simulink model "adc_sample"  (Simulink 8.3)
settings: Solver=ode5  StartTime=0.0  StopTime=3  FixedStep=1/20000  RelTol=1e-3
libraries: dsparch4 x2
settings Model: Creator=hlzhang  LastModifiedBy=hlzhang
settings DataIOCC: SignalLoggingName=sigsOut
settings DebuggingCC: SaveWithParameterizedLinksMsg=none  SignalResolutionControl=TryResolveAllWithWarning  SolverPrmCheckMsg=none  MultiTaskDSMMsg=warning  MultiTaskCondExecSysMsg=none  StateNameClashWarn=none
settings HardwareCC: TargetUnknown=on
settings RTWCC: IncludeERTFirstTime=on

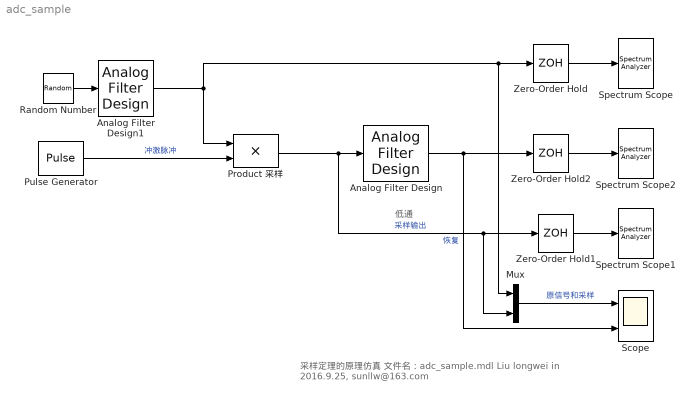
== system adc_sample ==
  note: 低通
  note: 采样定理的原理仿真
      | 文件名：adc_sample.mdl
      | Liu longwei in 2016.9.25, sunllw@163.com
  Analog Filter Design : dsparch4/Analog Filter Design  method=Butterworth  filttype=Lowpass  N=8  Wlo=2*pi*200  Whi=80  Rp=2  Rs=40
  Analog Filter Design1 : dsparch4/Analog Filter Design  method=Butterworth  filttype=Lowpass  N=50  Wlo=2*pi*250  Whi=80  Rp=2  Rs=40
  Mux : Mux  Inputs=2
  Product 采样 : Product  SaturateOnIntegerOverflow=on  OutDataTypeStr=Inherit: Same as first input
  Pulse Generator : DiscretePulseGenerator  Period=10  SampleTime=1/20000
  Random Number : RandomNumber  SampleTime=1/20000
  Scope : Scope  NumInputPorts=2
      settings: TimeRange=0.1  YMin=-0.8~-0.08  YMax=0.8~0.08
  Spectrum Scope : SpectrumAnalyzer  ScopeSpecification=DataTag0
  Spectrum Scope1 : SpectrumAnalyzer  ScopeSpecification=DataTag1
  Spectrum Scope2 : SpectrumAnalyzer  ScopeSpecification=DataTag2
  Zero-Order Hold : ZeroOrderHold  SampleTime=1/20000
  Zero-Order Hold1 : ZeroOrderHold  SampleTime=1/20000
  Zero-Order Hold2 : ZeroOrderHold  SampleTime=1/20000
  wires:
  Analog Filter Design1/1 -> Product 采样/1, Zero-Order Hold/1, Mux/1
  Pulse Generator/1 -> Product 采样/2  "冲激脉冲"
  Analog Filter Design/1 -> Zero-Order Hold2/1, Scope/2  "恢复"
  Zero-Order Hold/1 -> Spectrum Scope/1
  Zero-Order Hold1/1 -> Spectrum Scope1/1
  Zero-Order Hold2/1 -> Spectrum Scope2/1
  Random Number/1 -> Analog Filter Design1/1
  Product 采样/1 -> Analog Filter Design/1, Zero-Order Hold1/1, Mux/2  "采样输出"
  Mux/1 -> Scope/1  "原信号和采样"
